simulink model "pressure_controller_test_calibration"  (R2025b)
settings: Solver=FixedStepAuto  StartTime=0.0  StopTime=3  FixedStep=1e-3  RelTol=1e-3
model workspace (MAT data in the model file):
  Cmax = 0.912
  alpha = 55
  backlash = 0
  filter_freq = 0.0078
  manifold_bias = -57
  nozzle_bias = 0
undefined symbols (not defined in the file or in its folder): controllerGains
libraries: metux_library x2, eeGeneralControl x1
settings Model: Creator=karadeli  LastModifiedBy=karadeli

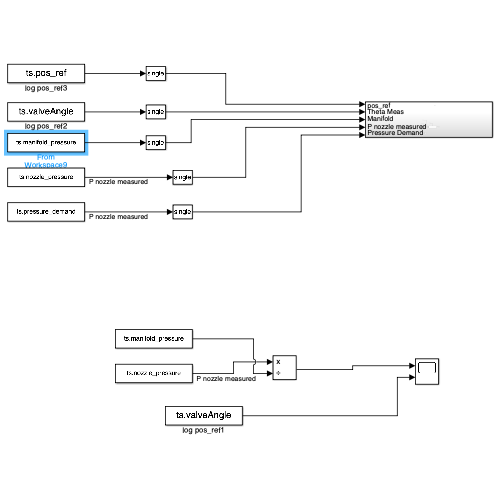
[thumbnail: Simulink's stored preview of the top-level diagram]
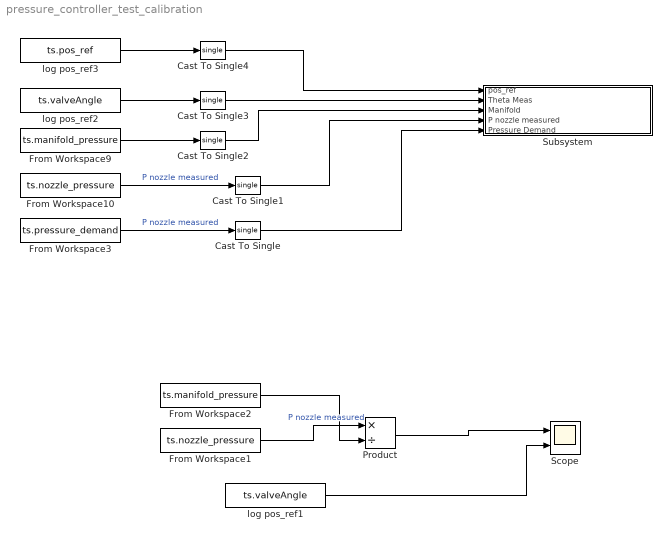
== system pressure_controller_test_calibration ==
  Cast To Single{,1..4} (5 alike) : DataTypeConversion  OutDataTypeStr=single  SaturateOnIntegerOverflow=off  RndMeth=Floor
  From Workspace1 : FromWorkspace  VariableName=ts.nozzle_pressure
  From Workspace10 : FromWorkspace  VariableName=ts.nozzle_pressure
  From Workspace2 : FromWorkspace  VariableName=ts.manifold_pressure
  From Workspace3 : FromWorkspace  VariableName=ts.pressure_demand
  From Workspace9 : FromWorkspace  VariableName=ts.manifold_pressure
  Product : Product  Inputs=*/
  Scope : Scope  NumInputPorts=2
      settings: ActiveDisplayYMinimum=-0.12175936523009334  ActiveDisplayYMaximum=0.29455323278843343
  Subsystem : Subsystem
  log pos_ref1 : FromWorkspace  VariableName=ts.valveAngle  Interpolate=off  OutputAfterFinalValue=Setting to zero
  log pos_ref2 : FromWorkspace  VariableName=ts.valveAngle  Interpolate=off  OutputAfterFinalValue=Setting to zero
  log pos_ref3 : FromWorkspace  VariableName=ts.pos_ref  Interpolate=off  OutputAfterFinalValue=Setting to zero
  wires:
  log pos_ref2/1 -> Cast To Single3/1
  From Workspace9/1 -> Cast To Single2/1
  From Workspace10/1 -> Cast To Single1/1  "P nozzle measured"
  From Workspace1/1 -> Product/1  "P nozzle measured"
  From Workspace2/1 -> Product/2
  Product/1 -> Scope/1
  log pos_ref1/1 -> Scope/2
  From Workspace3/1 -> Cast To Single/1  "P nozzle measured"
  log pos_ref3/1 -> Cast To Single4/1
  Cast To Single/1 -> Subsystem/5(Pressure Demand)
  Cast To Single1/1 -> Subsystem/4(P nozzle measured)
  Cast To Single2/1 -> Subsystem/3(Manifold)
  Cast To Single3/1 -> Subsystem/2(Theta Meas)
  Cast To Single4/1 -> Subsystem/1(pos_ref)

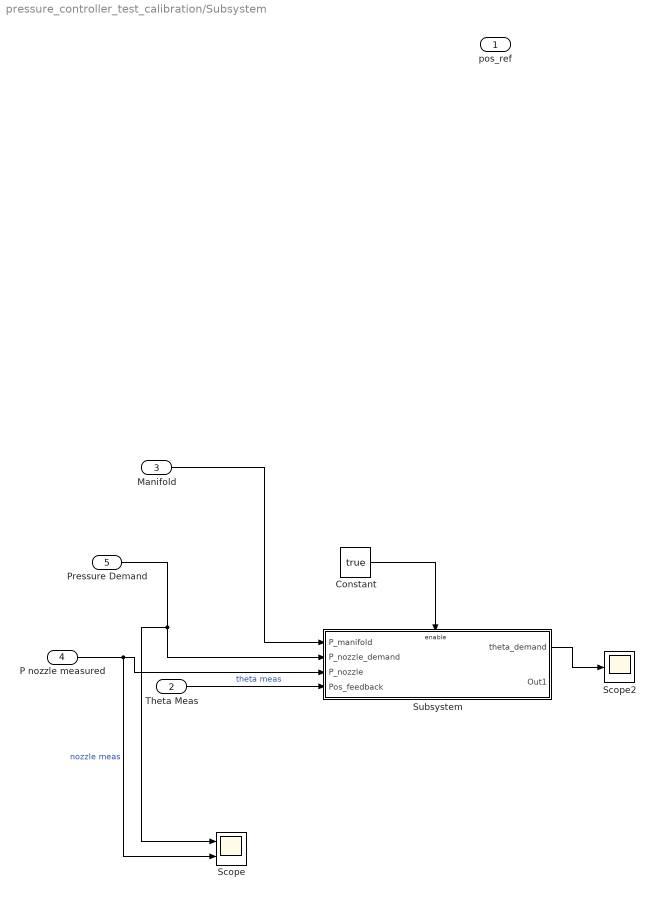
== system pressure_controller_test_calibration/Subsystem ==
  pos_ref : Inport
  Theta Meas : Inport  Port=2
  Manifold : Inport  Port=3
  P nozzle measured : Inport  Port=4
  Pressure Demand : Inport  Port=5
  Constant : Constant  Value=true
  Scope : Scope  NumInputPorts=2
      settings: ActiveDisplayYMinimum=-1  ActiveDisplayYMaximum=1  DataLoggingVariableName=ScopeData7
  Scope2 : Scope
      settings: ActiveDisplayYMinimum=-1  ActiveDisplayYMaximum=1  DataLoggingVariableName=ScopeData4
  Subsystem : Subsystem
  wires:
  Pressure Demand/1 -> Scope/1, Subsystem/2(P_nozzle_demand)
  Constant/1 -> Subsystem/Enable
  Theta Meas/1 -> Subsystem/4(Pos_feedback)  "theta meas"
  Manifold/1 -> Subsystem/1(P_manifold)
  P nozzle measured/1 -> Scope/2, Subsystem/3(P_nozzle)  "nozzle meas"
  Subsystem/1(theta_demand) -> Scope2/1

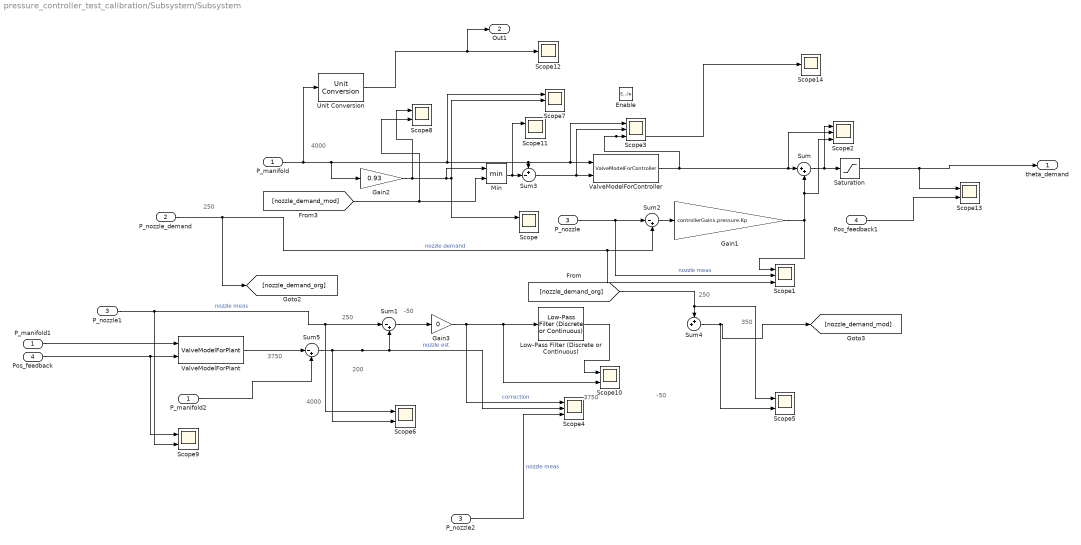
== system pressure_controller_test_calibration/Subsystem/Subsystem ==
  note: 250
  note: 3750
  note: 4000
  note: 3750
  note: 4000
  note: 200
  note: 250
  note: 250
  note: 350
  note: -50
  note: -50
  P_manifold : Inport  Unit=psi
  P_nozzle_demand : Inport  Port=2
  P_nozzle : Inport  Port=3
  Pos_feedback : Inport  Port=4
  Enable : EnablePort  StatesWhenEnabling=reset
  Gain1 : Gain  Gain=controllerGains.pressure.Kp
  Gain2 : Gain  Gain=0.93
  Gain3 : Gain  Gain=0
  Low-Pass Filter (Discrete or Continuous) : eeGeneralControl/Low-Pass Filter (Discrete or Continuous)  K=1  T=0.004  B=1000  A=-1000  init_option=Inherited from block input  x0=0  Ts=-1
  Min : MinMax  Inputs=2
  P_manifold1 : InportShadow  Unit=psi
  P_manifold2 : InportShadow  Unit=psi
  P_nozzle1 : InportShadow  Port=3
  P_nozzle2 : InportShadow  Port=3
  Pos_feedback1 : InportShadow  Port=4
  Saturation : Saturate  UpperLimit=1080  LowerLimit=0
  Scope{,5..6,8..11,13} (8 alike) : Scope  NumInputPorts=2
      Scope settings: ActiveDisplayYMinimum=-543.89154052734364  ActiveDisplayYMaximum=4895.0238647460938
      Scope10 settings: ActiveDisplayYMinimum=-1  ActiveDisplayYMaximum=1  DataLoggingVariableName=ScopeData12
      Scope11 settings: ActiveDisplayYMinimum=-93.749999999999986  ActiveDisplayYMaximum=843.75  DataLoggingVariableName=ScopeData13
      Scope13 settings: ActiveDisplayYMinimum=-37.528384021134109  ActiveDisplayYMaximum=337.647196748876  DataLoggingVariableName=ScopeData15
      Scope5 settings: ActiveDisplayYMinimum=-276.52408465355393  ActiveDisplayYMaximum=976.83862350828122  DataLoggingVariableName=ScopeData6
      Scope6 settings: ActiveDisplayYMinimum=-124.256647824087  ActiveDisplayYMaximum=995.51570772086041  DataLoggingVariableName=ScopeData8
      Scope8 settings: ActiveDisplayYMinimum=-1  ActiveDisplayYMaximum=1  DataLoggingVariableName=ScopeData10
      Scope9 settings: ActiveDisplayYMinimum=-1  ActiveDisplayYMaximum=1  DataLoggingVariableName=ScopeData11
  Scope{1..4,7} (5 alike) : Scope  NumInputPorts=3
      Scope1 settings: ActiveDisplayYMinimum=-1  ActiveDisplayYMaximum=1
      Scope2 settings: ActiveDisplayYMinimum=-238.99989700317383  ActiveDisplayYMaximum=406.84257888793945  DataLoggingVariableName=ScopeData2
      Scope3 settings: ActiveDisplayYMinimum=1655.9615783691406  ActiveDisplayYMaximum=3658.7408142089844  DataLoggingVariableName=ScopeData3
      Scope4 settings: ActiveDisplayYMinimum=-1  ActiveDisplayYMaximum=1  DataLoggingVariableName=ScopeData5
      Scope7 settings: ActiveDisplayYMinimum=-353.35925292968744  ActiveDisplayYMaximum=3180.2332763671875  DataLoggingVariableName=ScopeData9
  Scope12 : Scope
      settings: ActiveDisplayYMinimum=158.69168853759766  ActiveDisplayYMaximum=247.31496429443359  DataLoggingVariableName=ScopeData14
  Scope14 : Scope
      settings: ActiveDisplayYMinimum=-11.126747131347654  ActiveDisplayYMaximum=100.14072418212891  DataLoggingVariableName=ScopeData16
  Sum : Sum  Inputs=|++
  Sum1 : Sum  Inputs=|-+
  Sum2 : Sum  Inputs=|-+
  Sum3 : Sum  Inputs=+-|  OutDataTypeStr=single
  Sum4 : Sum  Inputs=++|
  Sum5 : Sum  Inputs=|-+
  Unit Conversion : UnitConversion
  ValveModelForController : metux_library/ValveModelForController  alpha=51.8534  C_max=0.9197
  ValveModelForPlant : metux_library/ValveModelForPlant  C_max=0.9197  alpha=51.8534
  theta_demand : Outport  OutputWhenDisabled=reset  InitialOutput=0
  Out1 : Outport  Port=2  Unit=bar
  wires:
  Saturation/1 -> Scope13/1, theta_demand/1
  Gain2/1 -> Scope8/1, Min/1, Scope7/2, Scope/1
  P_manifold/1 -> Unit Conversion/1, Sum3/1, Scope3/1, ValveModelForController/1, Scope7/1, Gain2/1
  P_nozzle_demand/1 -> [nozzle_demand_org], Scope1/3, Sum2/2  "nozzle demand"
  Sum3/1 -> Scope3/2, ValveModelForController/2
  P_nozzle/1 -> Scope1/2, Sum2/1  "nozzle meas"
  Gain1/1 -> Sum/2, Scope2/3, Scope1/1
  Sum/1 -> Scope2/1, Saturation/1
  Sum2/1 -> Gain1/1
  P_manifold1/1 -> ValveModelForPlant/1
  P_nozzle1/1 -> Scope9/2, Sum1/1, Scope6/1  "nozzle meas"
  ValveModelForPlant/1 -> Sum5/1
  [nozzle_demand_org] -> Scope5/1, Sum4/1
  Sum1/1 -> Gain3/1
  Gain3/1 -> Scope10/2, Low-Pass Filter (Discrete or Continuous)/1, Scope4/1  "correction"
  P_manifold2/1 -> Sum5/2
  Sum4/1 -> Scope5/2, [nozzle_demand_mod]
  [nozzle_demand_mod] -> Scope8/2, Min/2
  P_nozzle2/1 -> Scope4/3  "nozzle meas"
  Sum5/1 -> Scope4/2, Sum1/2, Scope6/2  "nozzle est"
  Min/1 -> Scope11/1, Sum3/2
  Low-Pass Filter (Discrete or Continuous)/1 -> Scope10/1
  Pos_feedback/1 -> Scope9/1, ValveModelForPlant/2
  Unit Conversion/1 -> Out1/1, Scope12/1
  Pos_feedback1/1 -> Scope13/2
  ValveModelForController/1 -> Scope14/1, Scope3/3, Scope2/2, Sum/1
